simulink model "Simulink_MPC_Main"  (R2023b)
settings: Solver=ode1  StartTime=0.0  StopTime=100  FixedStep=SampleTime  MaxStep=0.01  RelTol=1e-3  EnableMultiTasking=on
values from neighbouring files (symbols this model uses):
  Delay = 3    [Prepare_MPC_005.m]
  FilterDer0 = [8.542800360484532896e-02 ... (first row only)    [Prepare_MPC_005.m]
  FilterDer1 = [2.939212680227305530e+00 ... (first row only)    [Prepare_MPC_005.m]
  SampleTime = 0.05    [Prepare_MPC_005.m]
undefined symbols (not defined in the file or in its folder): GetPosition, length_trajectory_s, poly_approx_trajectory, UpdateBoard
libraries: sldrtlib x1
(part 2 of 2)

== matlab function Simulink_MPC_Main/SOLVE OCP /Nonlinear Model1/MATLAB Function4 ==
  data: x_in input; PWM input; x_end output; SampleTime input; Delay input
function x_end = Integrate_rk4(x_in, PWM,SampleTime,Delay)

% X_PWM_Simtime = PWM(1,:);
% Y_PWM_Simtime = PWM(2,:);
% Z_PWM_Simtime = PWM(3,:);
dt =  0.001; % Time step for RK4 integration
% nSteps = 451;
nSteps = Delay*(SampleTime/dt) +1;
Delay = ceil(Delay);
time_full = [0:dt:nSteps*dt-dt];
time_red = [0:SampleTime:Delay*SampleTime];
Signal = PWM(:,Delay+1:-1:1)
Signal_interp1 = interp1(time_red, Signal(1,:), time_full, 'previous');  % You can change 'linear' to other methods like 'spline', 'pchip', etc.
Signal_interp2 = interp1(time_red, Signal(2,:), time_full, 'previous');  % You can change 'linear' to other methods like 'spline', 'pchip', etc.

% l0 = 0.1712;
params = struct;
% Initialize output matrix for the RK4 results
% Apply coordinate transform to fit model
% x = [x_in(1) x_in(2) x_in(3)+l0  x_in(4) x_in(5) x_in(6) (x_in(7)) x_in(8) x_in(9) x_in(10)]; % Initial state
x = x_in';
% rk4Results = zeros(nSteps, length(x));
% rk4Results(1, :) = x_in'; % Initial state

for i = 1:nSteps-1
    % Current input
    u = [Signal_interp1(:,i) Signal_interp2(:,i) 0];
    % RK4 Integration
    k1 = crane3DModel_derivation(x, u);
    k2 = crane3DModel_derivation(x + 0.5*dt*k1, u);
    k3 = crane3DModel_derivation(x + 0.5*dt*k2, u);
    k4 = crane3DModel_derivation(x + dt*k3, u);
    
    x = x + dt*(k1 + 2*k2 + 2*k3 + k4)/6;
    % rk4Results(i+1, :) = [x(1), x(2), x(3)-l0,(x(4)), x(5) ,x(6), x(7), x(8), x(9), x(10)];
  % rk4Results(i+1, :) = x;

end
x_end = x;
end

== matlab function Simulink_MPC_Main/SOLVE OCP /Nonlinear Model1/MATLAB Function11 ==
  settings: updateMethod=DISCRETE
  data: u input; y output size=[3,7]
function y = CircularBuffer(u)
%#codegen
% Function to implement a simple N element circular buffer

% Define the internal buffer variable as persistent
persistent buffer
Initial_Buffer = ones(3, 7);

% Initialize the buffer the first time through
if isempty(buffer)
    % Initialize the buffer with the initial buffer
    buffer = zeros(3, 7);
    % Place the first input into the buffer
    buffer(:,1) = u;
else
    % Shift the buffer and insert the new input at the beginning
    buffer = [u, buffer(:,1:end-1)];
end

% Output the buffer
y = buffer;

end

== matlab function Simulink_MPC_Main/SOLVE OCP /Subsystem5/MPC 1/MATLAB Function3 ==
  data: x input; current output
function current = fcn(x)
current = [x(:,1)];

== matlab function Simulink_MPC_Main/SOLVE OCP /Subsystem4/MPC 1/MATLAB Function2 ==
  data: u input; u_warm output size=DimU
function u_warm = fcn(u)

u_warm = [u(:,2:end) u(:,end)];

== matlab function Simulink_MPC_Main/SOLVE OCP /Subsystem4/MPC 1/MATLAB Function3 ==
  data: x input; current output
function current = fcn(x)
current = [x(:,1)];

== matlab function Simulink_MPC_Main/SOLVE OCP /Subsystem4/MPC 1/Subsystem4/MATLAB Function8 ==
  data: traj input; first_elemt_traj output
function first_elemt_traj = getfirstelement(traj)

first_elemt_traj = traj(:,1);

== matlab function Simulink_MPC_Main/SOLVE OCP /Subsystem5/MPC 1/MATLAB Function4 ==
  data: u input; y output
function y = fcn(u)

y = u(1,1);

== matlab function Simulink_MPC_Main/SOLVE OCP /Subsystem5/MPC 1/MATLAB Function5 ==
  data: x input; current output
function current = fcn(x)
current = [x(:,1)];

== matlab function Simulink_MPC_Main/Subsystem1/Subsystem/Subsystem5/Subsystem1/MATLAB Function11 ==
  settings: updateMethod=DISCRETE
  data: u input; y output size=[1,N_Coeff]; Initial_Buffer input
function y = CircularBuffer(u,Initial_Buffer)
%#codegen
% Function to implement a simple N element circular buffer

% Define the internal buffer variable as persistent
persistent buffer



% Initialize the buffer the first time through
if isempty(buffer)
    % Initialize the buffer
    buffer = Initial_Buffer*u;
    % buff_entrys = 1;
    buffer(1) = u;
else
    % wenn nicht leer, dann schiebe eins hoch 
    buff2 = buffer; 
    buffer = [u; buff2(1:end-1)];
end

% Output the buffer
y = buffer';

end

== matlab function Simulink_MPC_Main/SOLVE OCP /Subsystem5/Trajectroy ==
  data: coeffs input; evaluated_polynomials_X output; t input size=[1 1]
function evaluated_polynomials_X = evaluatePolynomials(coeffs, t)


    % % Initialize an array to hold the evaluated polynomials
    num_trajectories = size(coeffs, 1); % Number of trajectories (rows of coeffs)
    % evaluated_polynomials = casadi.MX(num_trajectories, 1);
     evaluated_polynomials = zeros(num_trajectories, 1);
    % 
    % Loop over each set of coefficients (each trajectory)
    for j = 1:num_trajectories
        % Get the coefficients for this trajectory
        current_coeffs = coeffs(j, :);
        % Find the degree of the polynomial based on the number of coefficients
        degree = length(current_coeffs) - 1;

        % Initialize the polynomial expression to zero for this trajectory
        % current_polynomial = casadi.MX(1,1);
        current_polynomial = zeros(1,1);
        % Evaluate the polynomial using a loop, considering the order of coefficients
        for i = 0:degree
            % Add each term of the polynomial
            current_polynomial = current_polynomial + current_coeffs(degree + 1 - i) * t^i;
        end

        % Evaluate the current polynomial at the given time t
        evaluated_polynomials(j) = (current_polynomial);
    end
    if num_trajectories ==8
    % evaluated_polynomials(1) = 0.25 + 0.2*sin(t);
    % evaluated_polynomials(2) = 0.25 + 0.2*cos(t);
    % evaluated_polynomials(3) = 0;
    % evaluated_polynomials(3:8) = zeros(6,1);
    else
        % evaluated_polynomials = zeros(2,1);
    end
    evaluated_polynomials_X = evaluated_polynomials([1,3,5,7]);
end

== matlab function Simulink_MPC_Main/SOLVE OCP /Subsystem1/MATLAB Function3 ==
  data: u input; u_plant output size=[1,1]; x input; x_new output
function [u_plant,x_new] = fcn(u,x)

x_new = x(:,2);
u_plant = u(:,1);

== matlab function Simulink_MPC_Main/SOLVE OCP /Subsystem1/MPC 1/MATLAB Function ==
  data: x input; x_warm output
function x_warm = fcn(x)
x_warm = [x(:,3:end) x(:,end)];

== matlab function Simulink_MPC_Main/SOLVE OCP /Subsystem1/MPC 1/MATLAB Function1 ==
  data: lam_g input; lam_g_warm output
function lam_g_warm = fcn(lam_g)
lam_g_warm = lam_g;

== matlab function Simulink_MPC_Main/SOLVE OCP /Subsystem1/MPC 1/MATLAB Function2 ==
  data: u input; u_warm output size=DimU
function u_warm = fcn(u)

u_warm = [u(:,2:end) u(:,end)];

== matlab function Simulink_MPC_Main/SOLVE OCP /Subsystem1/MPC 1/MATLAB Function3 ==
  data: x input; current output
function current = fcn(x)
current = [x(:,1)];

== matlab function Simulink_MPC_Main/SOLVE OCP /Subsystem1/MPC 1/MATLAB Function4 ==
  data: u input; y output
function y = fcn(u)

y = u(1,1);

== matlab function Simulink_MPC_Main/SOLVE OCP /Subsystem1/MPC 1/MATLAB Function5 ==
  data: x input; current output
function current = fcn(x)
current = [x(:,1)];

== matlab function Simulink_MPC_Main/SOLVE OCP /Subsystem1/MPC 1/Subsystem4/MATLAB Function8 ==
  data: traj input; first_elemt_traj output
function first_elemt_traj = getfirstelement(traj)

first_elemt_traj = traj(:,1);

== matlab function Simulink_MPC_Main/SOLVE OCP /Subsystem1/Trajectroy ==
  data: coeffs input; evaluated_polynomials_X output; t input size=[1 1]
function evaluated_polynomials_X = evaluatePolynomials(coeffs, t)


    % % Initialize an array to hold the evaluated polynomials
    num_trajectories = size(coeffs, 1); % Number of trajectories (rows of coeffs)
    % evaluated_polynomials = casadi.MX(num_trajectories, 1);
     evaluated_polynomials = zeros(num_trajectories, 1);
    % 
    % Loop over each set of coefficients (each trajectory)
    for j = 1:num_trajectories
        % Get the coefficients for this trajectory
        current_coeffs = coeffs(j, :);
        % Find the degree of the polynomial based on the number of coefficients
        degree = length(current_coeffs) - 1;

        % Initialize the polynomial expression to zero for this trajectory
        % current_polynomial = casadi.MX(1,1);
        current_polynomial = zeros(1,1);
        % Evaluate the polynomial using a loop, considering the order of coefficients
        for i = 0:degree
            % Add each term of the polynomial
            current_polynomial = current_polynomial + current_coeffs(degree + 1 - i) * t^i;
        end

        % Evaluate the current polynomial at the given time t
        evaluated_polynomials(j) = (current_polynomial);
    end
    if num_trajectories ==8
    % evaluated_polynomials(1) = 0.25 + 0.2*sin(t);
    % evaluated_polynomials(2) = 0.25 + 0.2*cos(t);
    % evaluated_polynomials(3) = 0;
    % evaluated_polynomials(3:8) = zeros(6,1);
    else
        % evaluated_polynomials = zeros(2,1);
    end
    evaluated_polynomials_X = evaluated_polynomials([1,3,5,7]);
end

== matlab function Simulink_MPC_Main/Subsystem1/Subsystem/Subsystem5/Subsystem2/MATLAB Function11 ==
  settings: updateMethod=DISCRETE
  data: u input; y output size=[1,N_Coeff]; Initial_Buffer input
function y = CircularBuffer(u,Initial_Buffer)
%#codegen
% Function to implement a simple N element circular buffer

% Define the internal buffer variable as persistent
persistent buffer



% Initialize the buffer the first time through
if isempty(buffer)
    % Initialize the buffer
    buffer = Initial_Buffer*u;
    % buff_entrys = 1;
    buffer(1) = u;
else
    % wenn nicht leer, dann schiebe eins hoch 
    buff2 = buffer; 
    buffer = [u; buff2(1:end-1)];
end

% Output the buffer
y = buffer';

end

== matlab function Simulink_MPC_Main/MATLAB Function ==
  data: u input; u output; t input; enable input
function u  = disturbance(u, t,enable)
if ~enable
u = u;
else
    % Define the time intervals for disturbances
    Time_Disturbance1 = [20, 23];
    Time_Disturbance2 = [40, 41];
    Time_Disturbance3 = [58, 60];
    Time_Disturbance4 = [80, 90];

    % Determine which disturbance interval t falls into
    if t >= min(Time_Disturbance1) && t <= max(Time_Disturbance1)
        current_Disturbance = 'Time_Disturbance1';
    elseif t >= min(Time_Disturbance2) && t <= max(Time_Disturbance2)
        current_Disturbance = 'Time_Disturbance2';
    elseif t >= min(Time_Disturbance3) && t <= max(Time_Disturbance3)
        current_Disturbance = 'Time_Disturbance3';
    elseif t >= min(Time_Disturbance4) && t <= max(Time_Disturbance4)
        current_Disturbance = 'Time_Disturbance4';
    else
        current_Disturbance = 'None';
    end

    % Switch statement based on the current disturbance
    switch current_Disturbance
        case 'Time_Disturbance1'

        u = ones(2,1);
        case 'Time_Disturbance2'

            u = zeros(2,1);


        case 'Time_Disturbance3'
u(1) = -1*sin(3*t);
u(2) = 0 ;
        case 'Time_Disturbance4'
       u(1) = u(1) + 0.4*sin(4*t);
u(2) = u(2) + 0.4*sin(5*t); 
        otherwise

    end
end
end

== matlab function Simulink_MPC_Main/SOLVE OCP /Subsystem2/Delete L ==
  data: x10 input; x_8 output
function x_8 = fcn(x10)
relevantstates = [1,2,4,5,6,7,9,10];
x_8 =x10(relevantstates);

== matlab function Simulink_MPC_Main/SOLVE OCP /Subsystem2/MATLAB Function10 ==
  data: x_18 input; x_X output; x_Y output
function [x_X,x_Y] = add_int(x_18)
x_X = zeros(4,1);
x_Y = zeros(4,1);
x_X(1) = x_18(1);
x_Y(1) = x_18(2);
x_X(2) = x_18(3);
x_Y(2) = x_18(4);
x_X(3) = x_18(5);
x_Y(3) = x_18(6);
x_X(4) = x_18(7);
x_Y(4) = x_18(8);

== matlab function Simulink_MPC_Main/Subsystem1/Subsystem/Subsystem5/Subsystem3/MATLAB Function11 ==
  settings: updateMethod=DISCRETE
  data: u input; y output size=[1,N_Coeff]; Initial_Buffer input
function y = CircularBuffer(u,Initial_Buffer)
%#codegen
% Function to implement a simple N element circular buffer

% Define the internal buffer variable as persistent
persistent buffer



% Initialize the buffer the first time through
if isempty(buffer)
    % Initialize the buffer
    buffer = Initial_Buffer*u;
    % buff_entrys = 1;
    buffer(1) = u;
else
    % wenn nicht leer, dann schiebe eins hoch 
    buff2 = buffer; 
    buffer = [u; buff2(1:end-1)];
end

% Output the buffer
y = buffer';

end

== matlab function Simulink_MPC_Main/Subsystem1/Subsystem/Subsystem5/Subsystem4/MATLAB Function11 ==
  settings: updateMethod=DISCRETE
  data: u input; y output size=[1,N_Coeff]; Initial_Buffer input
function y = CircularBuffer(u,Initial_Buffer)
%#codegen
% Function to implement a simple N element circular buffer

% Define the internal buffer variable as persistent
persistent buffer



% Initialize the buffer the first time through
if isempty(buffer)
    % Initialize the buffer
    buffer = Initial_Buffer*u;
    % buff_entrys = 1;
    buffer(1) = u;
else
    % wenn nicht leer, dann schiebe eins hoch 
    buff2 = buffer; 
    buffer = [u; buff2(1:end-1)];
end

% Output the buffer
y = buffer';

end

== matlab function Simulink_MPC_Main/Subsystem1/Subsystem/Subsystem5/Subsystem10/MATLAB Function11 ==
  settings: updateMethod=DISCRETE
  data: u input; y output size=[1,N_Coeff]; Initial_Buffer input
function y = CircularBuffer(u,Initial_Buffer)
%#codegen
% Function to implement a simple N element circular buffer

% Define the internal buffer variable as persistent
persistent buffer



% Initialize the buffer the first time through
if isempty(buffer)
    % Initialize the buffer
    buffer = Initial_Buffer*u;
    % buff_entrys = 1;
    buffer(1) = u;
else
    % wenn nicht leer, dann schiebe eins hoch 
    buff2 = buffer; 
    buffer = [u; buff2(1:end-1)];
end

% Output the buffer
y = buffer';

end

== matlab function Simulink_MPC_Main/Subsystem1/Subsystem/Subsystem5/Subsystem11/MATLAB Function11 ==
  settings: updateMethod=DISCRETE
  data: u input; y output size=[1,N_Coeff]; Initial_Buffer input
function y = CircularBuffer(u,Initial_Buffer)
%#codegen
% Function to implement a simple N element circular buffer

% Define the internal buffer variable as persistent
persistent buffer



% Initialize the buffer the first time through
if isempty(buffer)
    % Initialize the buffer
    buffer = Initial_Buffer*u;
    % buff_entrys = 1;
    buffer(1) = u;
else
    % wenn nicht leer, dann schiebe eins hoch 
    buff2 = buffer; 
    buffer = [u; buff2(1:end-1)];
end

% Output the buffer
y = buffer';

end

== matlab function Simulink_MPC_Main/Subsystem1/Subsystem/Subsystem5/Subsystem12/MATLAB Function11 ==
  settings: updateMethod=DISCRETE
  data: u input; y output size=[1,N_Coeff]; Initial_Buffer input
function y = CircularBuffer(u,Initial_Buffer)
%#codegen
% Function to implement a simple N element circular buffer

% Define the internal buffer variable as persistent
persistent buffer



% Initialize the buffer the first time through
if isempty(buffer)
    % Initialize the buffer
    buffer = Initial_Buffer*u;
    % buff_entrys = 1;
    buffer(1) = u;
else
    % wenn nicht leer, dann schiebe eins hoch 
    buff2 = buffer; 
    buffer = [u; buff2(1:end-1)];
end

% Output the buffer
y = buffer';

end

== matlab function Simulink_MPC_Main/Subsystem1/Subsystem/Subsystem5/Subsystem13/MATLAB Function11 ==
  settings: updateMethod=DISCRETE
  data: u input; y output size=[1,N_Coeff]; Initial_Buffer input
function y = CircularBuffer(u,Initial_Buffer)
%#codegen
% Function to implement a simple N element circular buffer

% Define the internal buffer variable as persistent
persistent buffer



% Initialize the buffer the first time through
if isempty(buffer)
    % Initialize the buffer
    buffer = Initial_Buffer*u;
    % buff_entrys = 1;
    buffer(1) = u;
else
    % wenn nicht leer, dann schiebe eins hoch 
    buff2 = buffer; 
    buffer = [u; buff2(1:end-1)];
end

% Output the buffer
y = buffer';

end

== matlab function Simulink_MPC_Main/Subsystem1/Subsystem/Subsystem5/Subsystem14/MATLAB Function11 ==
  settings: updateMethod=DISCRETE
  data: u input; y output size=[1,N_Coeff]; Initial_Buffer input
function y = CircularBuffer(u,Initial_Buffer)
%#codegen
% Function to implement a simple N element circular buffer

% Define the internal buffer variable as persistent
persistent buffer



% Initialize the buffer the first time through
if isempty(buffer)
    % Initialize the buffer
    buffer = Initial_Buffer*u;
    % buff_entrys = 1;
    buffer(1) = u;
else
    % wenn nicht leer, dann schiebe eins hoch 
    buff2 = buffer; 
    buffer = [u; buff2(1:end-1)];
end

% Output the buffer
y = buffer';

end
